simulink library "csu_pbp_piksi_baseline_packet_lib"  (R2014b)
settings: Solver=ode45  StartTime=0.0  StopTime=10.0  RelTol=1e-3
undefined symbols (not defined in the file): gps_base_station_topocentric, gps_enu_to_ned_dcm, gps_jump_seed, gps_normal_rv_jump_limit, gps_rate_to_noise_std
libraries: util_common_lib x6, simulink x2, util_info_lib x1, util_frame_rotation_lib x1
settings Model: Creator=escrane  LastModifiedBy=mstewart

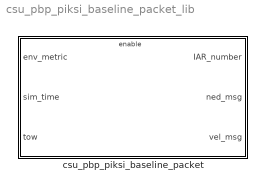
== system csu_pbp_piksi_baseline_packet_lib ==
  csu_pbp_piksi_baseline_packet : Subsystem

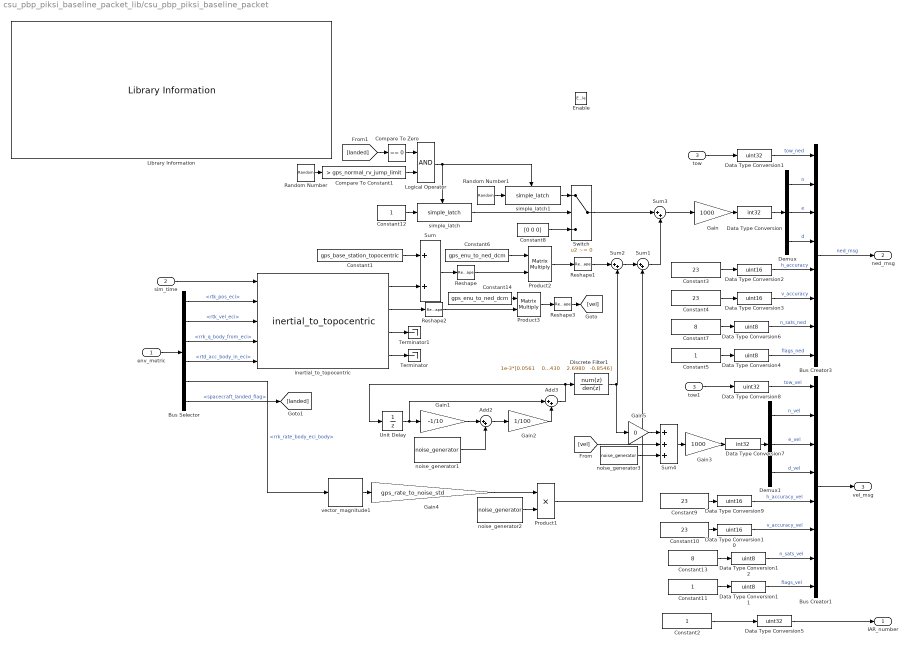
== system csu_pbp_piksi_baseline_packet_lib/csu_pbp_piksi_baseline_packet ==
  env_metric : Inport
  sim_time : Inport  Port=2
  tow : Inport  Port=3
  Enable : EnablePort
  Add2 : Sum  Inputs=|++
  Add3 : Sum  Inputs=|++
  Bus Creator1 : BusCreator  Inputs=8
  Bus Creator3 : BusCreator  Inputs=8
  Bus Selector : BusSelector  OutputSignals=lander_state_bus.rtk_pos_eci,lander_state_bus.rtk_vel_eci,lander_state_bus.rrk_q_body_from_eci,lander_state_bus.rtd_acc_body_in_eci,lander_state_bus.rrk_rate_body_eci_body,lander_state_bus.spacecraft_landed_flag
  Compare To Constant1 : simulink/Logic and Bit Operations/Compare To Constant  relop=>  const=gps_normal_rv_jump_limit  OutDataTypeStr=boolean
  Compare To Zero : simulink/Logic and Bit Operations/Compare To Zero  relop===  OutDataTypeStr=boolean
  Constant1 : Constant  Value=gps_base_station_topocentric
  Constant{3..4,9..10} (4 alike) : Constant  Value=23  OutDataTypeStr=double
  Constant{2,5,11..12} (4 alike) : Constant  OutDataTypeStr=double
  Constant13 : Constant  Value=8  OutDataTypeStr=double
  Constant14 : Constant  Value=gps_enu_to_ned_dcm
  Constant6 : Constant  Value=gps_enu_to_ned_dcm
  Constant7 : Constant  Value=8  OutDataTypeStr=double
  Constant8 : Constant  Value=[0 0 0]  OutDataTypeStr=double
  Data Type Conversion : DataTypeConversion  OutDataTypeStr=int32
  Data Type Conversion1 : DataTypeConversion  OutDataTypeStr=uint32
  Data Type Conversion{2..3,9..10} (4 alike) : DataTypeConversion  OutDataTypeStr=uint16
  Data Type Conversion{4,6,11..12} (4 alike) : DataTypeConversion  OutDataTypeStr=uint8
  Data Type Conversion5 : DataTypeConversion  OutDataTypeStr=uint32
  Data Type Conversion7 : DataTypeConversion  OutDataTypeStr=int32
  Data Type Conversion8 : DataTypeConversion  OutDataTypeStr=uint32
  Demux : Demux  Outputs=3
  Demux1 : Demux  Outputs=3
  Discrete Filter1 : DiscreteFilter  Numerator="1e-3*[0.0561    0.1682    0.1682    0.0561]"  Denominator="[1.0000   -2.8430    2.6980   -0.8546]"
  Gain : Gain  Gain=1000
  Gain1 : Gain  Gain=-1/10
  Gain2 : Gain  Gain=1/100
  Gain3 : Gain  Gain=1000
  Gain4 : Gain  Gain=gps_rate_to_noise_std
  Gain5 : Gain  Gain=0
  Library Information : util_info_lib/Library Information  owner='escrane'
  Logical Operator : Logic  AllPortsSameDT=off  OutDataTypeStr=boolean
  Product1 : Product
  Product2 : Product  Multiplication=Matrix(*)
  Product3 : Product  Multiplication=Matrix(*)
  Random Number : RandomNumber  Seed=gps_jump_seed  SampleTime=0.01
  Random Number1 : RandomNumber  Mean=[0 0 0]  Variance=[0.25 0.25 0.25]  Seed=[24 5 17]  SampleTime=0.01
  Reshape : Reshape  OutputDimensionality=Column vector (2-D)
  Reshape1 : Reshape
  Reshape2 : Reshape  OutputDimensionality=Column vector (2-D)
  Reshape3 : Reshape
  Sum : Sum
  Sum1 : Sum  Inputs=|++
  Sum2 : Sum  Inputs=|++
  Sum3 : Sum  Inputs=|++
  Sum4 : Sum  Inputs=+++
  Switch : Switch  Criteria=u2 ~= 0
  Terminator : Terminator
  Terminator1 : Terminator
  Unit Delay : UnitDelay  SampleTime=-1
  inertial_to_topocentric : util_frame_rotation_lib/inertial_to_topocentric  SystemSampleTime=-1
  noise_generator1 : util_common_lib/noise_generator  std_dev=gps_walk_noise_meters_std  bias=gps_walk_bias_meters  seed=gps_walk_noise_seed_number  on=gps_walk_noise_on  sample_time=sim_time_step_size
  noise_generator2 : util_common_lib/noise_generator  std_dev=1  bias=0  seed=gps_noise_seed_number  on=gps_noise_on  sample_time=sim_time_step_size
  noise_generator3 : util_common_lib/noise_generator  std_dev=0.16*[1 1 3]  bias=[0 0 0]  seed=gps_noise_seed_number  on=gps_noise_on  sample_time=sim_time_step_size
  simple_latch : util_common_lib/simple_latch  SystemSampleTime=-1
  simple_latch1 : util_common_lib/simple_latch  SystemSampleTime=-1
  tow1 : InportShadow  Port=3
  vector_magnitude1 : util_common_lib/vector_magnitude  SystemSampleTime=-1
  IAR_number : Outport
  ned_msg : Outport  Port=2
  vel_msg : Outport  Port=3
  wires:
  Compare To Zero/1 -> Logical Operator/1
  Compare To Constant1/1 -> Logical Operator/2
  [landed] -> Compare To Zero/1
  Bus Selector/6 -> [landed]  "<spacecraft_landed_flag>"
  noise_generator3/1 -> Sum4/3
  Gain5/1 -> Sum4/1
  [vel] -> Sum4/2
  Sum4/1 -> Gain3/1
  Reshape3/1 -> [vel]
  inertial_to_topocentric/2 -> Reshape2/1
  Product3/1 -> Reshape3/1
  Constant14/1 -> Product3/1
  Reshape2/1 -> Product3/2
  Bus Creator1/1 -> vel_msg/1
  Data Type Conversion12/1 -> Bus Creator1/7  "n_sats_vel"
  Constant13/1 -> Data Type Conversion12/1
  Data Type Conversion11/1 -> Bus Creator1/8  "flags_vel"
  Constant11/1 -> Data Type Conversion11/1
  Data Type Conversion10/1 -> Bus Creator1/6  "v_accuracy_vel"
  Constant10/1 -> Data Type Conversion10/1
  Data Type Conversion9/1 -> Bus Creator1/5  "h_accuracy_vel"
  Constant9/1 -> Data Type Conversion9/1
  Data Type Conversion8/1 -> Bus Creator1/1  "tow_vel"
  tow1/1 -> Data Type Conversion8/1
  Demux1/3 -> Bus Creator1/4  "d_vel"
  Demux1/2 -> Bus Creator1/3  "e_vel"
  Demux1/1 -> Bus Creator1/2  "n_vel"
  Data Type Conversion7/1 -> Demux1/1
  Gain3/1 -> Data Type Conversion7/1
  Switch/1 -> Sum3/1
  Sum3/1 -> Gain/1
  Sum1/1 -> Sum3/2
  Random Number1/1 -> simple_latch1/1
  Constant12/1 -> simple_latch/1
  simple_latch/1 -> Switch/2
  Random Number/1 -> Compare To Constant1/1
  simple_latch1/1 -> Switch/1
  Constant8/1 -> Switch/3
  Logical Operator/1 -> simple_latch1/Trigger, simple_latch/Trigger
  Product1/1 -> Sum1/2
  Data Type Conversion6/1 -> Bus Creator3/7  "n_sats_ned"
  Constant7/1 -> Data Type Conversion6/1
  Bus Creator3/1 -> ned_msg/1  "ned_msg"
  Data Type Conversion4/1 -> Bus Creator3/8  "flags_ned"
  Constant5/1 -> Data Type Conversion4/1
  Data Type Conversion3/1 -> Bus Creator3/6  "v_accuracy"
  Constant4/1 -> Data Type Conversion3/1
  Data Type Conversion2/1 -> Bus Creator3/5  "h_accuracy"
  Constant3/1 -> Data Type Conversion2/1
  Data Type Conversion1/1 -> Bus Creator3/1  "tow_ned"
  tow/1 -> Data Type Conversion1/1
  Demux/3 -> Bus Creator3/4  "d"
  Demux/2 -> Bus Creator3/3  "e"
  Demux/1 -> Bus Creator3/2  "n"
  Data Type Conversion/1 -> Demux/1
  inertial_to_topocentric/3 -> Terminator1/1
  inertial_to_topocentric/4 -> Terminator/1
  sim_time/1 -> inertial_to_topocentric/1
  env_metric/1 -> Bus Selector/1
  noise_generator1/1 -> Add2/2
  Gain1/1 -> Add2/1
  Add3/1 -> Unit Delay/1, Discrete Filter1/1
  Unit Delay/1 -> Add3/1, Gain1/1
  Gain2/1 -> Add3/2
  Add2/1 -> Gain2/1
  Bus Selector/4 -> inertial_to_topocentric/5  "<rtd_acc_body_in_eci>"
  Bus Selector/3 -> inertial_to_topocentric/4  "<rrk_q_body_from_eci>"
  Bus Selector/2 -> inertial_to_topocentric/3  "<rtk_vel_eci>"
  Bus Selector/1 -> inertial_to_topocentric/2  "<rtk_pos_eci>"
  Sum2/1 -> Sum1/1
  Constant1/1 -> Sum/1
  inertial_to_topocentric/1 -> Sum/2
  vector_magnitude1/1 -> Gain4/1
  Gain4/1 -> Product1/1
  noise_generator2/1 -> Product1/2
  Bus Selector/5 -> vector_magnitude1/1  "<rrk_rate_body_eci_body>"
  Sum/1 -> Reshape/1
  Product2/1 -> Reshape1/1
  Constant6/1 -> Product2/1
  Reshape/1 -> Product2/2
  Reshape1/1 -> Sum2/1
  Discrete Filter1/1 -> Sum2/2, Gain5/1
  Constant2/1 -> Data Type Conversion5/1
  Data Type Conversion5/1 -> IAR_number/1
  Gain/1 -> Data Type Conversion/1
